simulink model "lr_11"  (R2014b)
settings: Solver=ode45  StartTime=0.0  StopTime=20  MaxStep=0.001  RelTol=1e-3
settings Model: Creator=maksimka  LastModifiedBy=maksimka

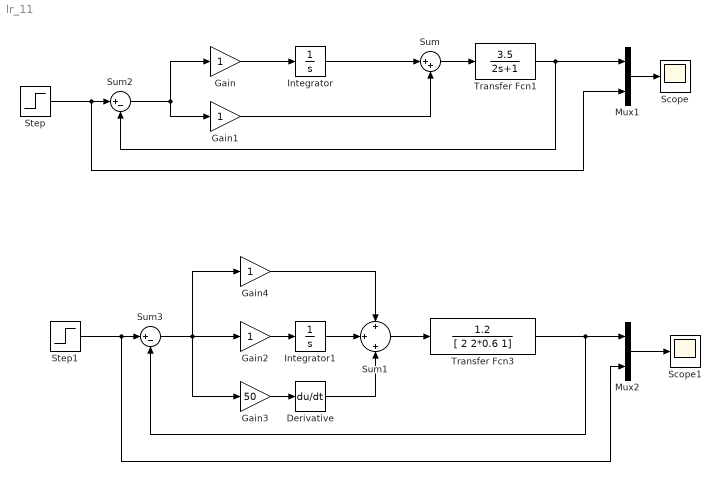
== system lr_11 ==
  Derivative : Derivative
  Gain{,1..2,4} (4 alike) : Gain
  Gain3 : Gain  Gain=50
  Integrator : Integrator
  Integrator1 : Integrator
  Mux1 : Mux  Inputs=2
  Mux2 : Mux  Inputs=2
  Scope : Scope
      settings: TimeRange=20  YMin=-1  YMax=1  MaxDataPoints=50000
  Scope1 : Scope
      settings: TimeRange=49.998322373481  YMin=0.9999999997000001  YMax=1.0000000001  MaxDataPoints=1000
  Step : Step  SampleTime=0
  Step1 : Step  SampleTime=0
  Sum : Sum  Inputs=|++
  Sum1 : Sum  Inputs=+|+|+
  Sum2 : Sum  Inputs=|+-
  Sum3 : Sum  Inputs=|+-
  Transfer Fcn1 : TransferFcn  Numerator=[3.5]  Denominator=[2 1]
  Transfer Fcn3 : TransferFcn  Numerator=[1.2]  Denominator=[ 2 2*0.6 1]
  wires:
  Sum2/1 -> Gain/1, Gain1/1
  Step/1 -> Mux1/2, Sum2/1
  Gain/1 -> Integrator/1
  Integrator/1 -> Sum/1
  Gain1/1 -> Sum/2
  Sum/1 -> Transfer Fcn1/1
  Transfer Fcn1/1 -> Sum2/2, Mux1/1
  Mux1/1 -> Scope/1
  Sum3/1 -> Gain2/1, Gain4/1, Gain3/1
  Step1/1 -> Mux2/2, Sum3/1
  Gain2/1 -> Integrator1/1
  Integrator1/1 -> Sum1/2
  Gain3/1 -> Derivative/1
  Sum1/1 -> Transfer Fcn3/1
  Mux2/1 -> Scope1/1
  Gain4/1 -> Sum1/1
  Derivative/1 -> Sum1/3
  Transfer Fcn3/1 -> Mux2/1, Sum3/2
